simulink model "Subsystem"  (R2018a)
settings: Solver=VariableStepAuto  StartTime=0.0  StopTime=5  RelTol=1e-3
settings Model: Creator=Ducted Fan  LastModifiedBy=Ducted Fan
settings SolverCC: ZeroCrossAlgorithm=Adaptive
settings DataIOCC: SaveOutput=off  SaveTime=off
settings DebuggingCC: MaxConsecutiveZCsMsg=none  MaskedZcDiagnostic=none  IgnoredZcDiagnostic=none

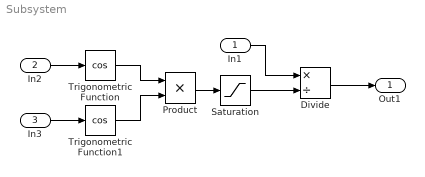
== system Subsystem ==
  In1 : Inport  OutDataTypeStr=double  PortDimensions=1
  In2 : Inport  Port=2  OutDataTypeStr=double  PortDimensions=1
  In3 : Inport  Port=3  OutDataTypeStr=double  PortDimensions=1
  Divide : Product  Inputs=*/
  Product : Product
  Saturation : Saturate  UpperLimit=1  LowerLimit=0.5
  Trigonometric Function : Trigonometry  Operator=cos
  Trigonometric Function1 : Trigonometry  Operator=cos
  Out1 : Outport  OutDataTypeStr=double  PortDimensions=1
  wires:
  In2/1 -> Trigonometric Function/1
  In3/1 -> Trigonometric Function1/1
  Trigonometric Function/1 -> Product/1
  Trigonometric Function1/1 -> Product/2
  Product/1 -> Saturation/1
  In1/1 -> Divide/1
  Saturation/1 -> Divide/2
  Divide/1 -> Out1/1
